simulink model "adc"  (R2024a)
settings: configuration reference "standardSILConfiguraitonParams" (kept outside this file)
undefined symbols (not defined in the file): stepSize_s
libraries: simulink x2, aerolibatmos2 x1
settings Model: Creator=GTAR  LastModifiedBy=jerem
settings ConfigSetRef: SourceName=standardSILConfiguraitonParams  SourceLocation=Base Workspace

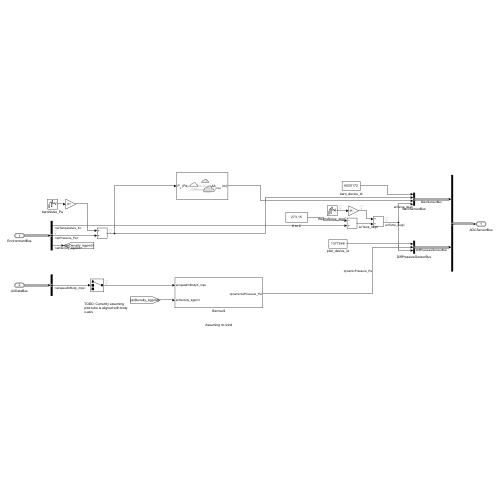
[thumbnail: Simulink's stored preview of the top-level diagram]
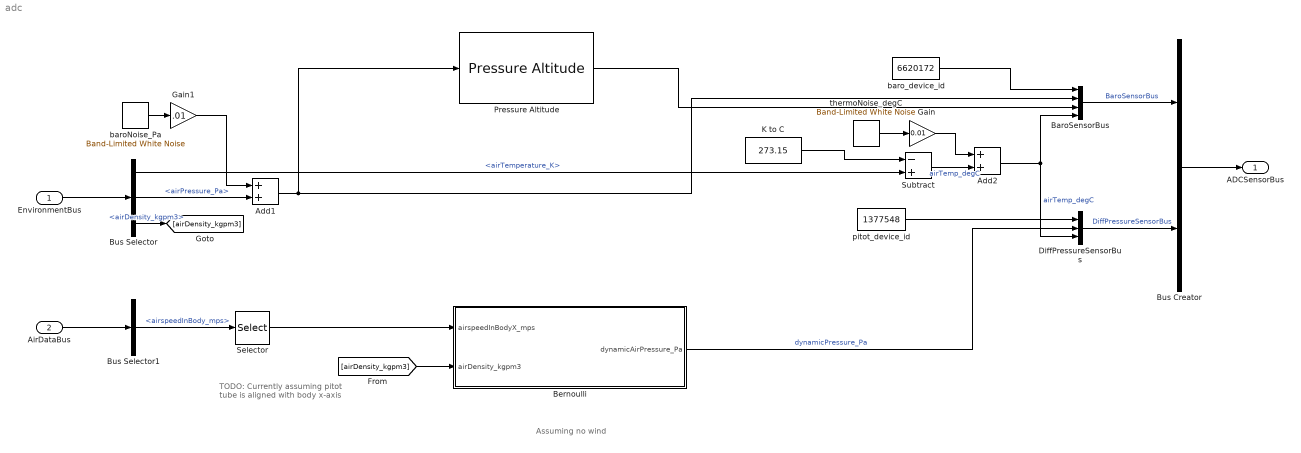
== system adc ==
  note: Assuming no wind
  note: TODO: Currently assuming pitot tube is aligned with body x-axis
  EnvironmentBus : Inport  OutDataTypeStr=Bus: EnvironmentBus
  AirDataBus : Inport  Port=2  OutDataTypeStr=Bus: AirData
  Add1 : Sum
  Add2 : Sum
  BaroSensorBus : BusCreator  Inputs=4  OutDataTypeStr=Bus: BaroSensorBus
      settings: InheritFromInputs=off
  Bernoulli : Subsystem
  Bus Creator : BusCreator  Inputs=2  OutDataTypeStr=Bus: ADCSensorBus
      settings: InheritFromInputs=off
  Bus Selector : BusSelector  OutputSignals=AirEnvironment.airTemperature_K,AirEnvironment.airPressure_Pa,AirEnvironment.airDensity_kgpm3
  Bus Selector1 : BusSelector  OutputSignals=airspeedInBody_mps
  DiffPressureSensorBus : BusCreator  Inputs=3  OutDataTypeStr=Bus: DiffPressureSensorBus
      settings: InheritFromInputs=off
  Gain : Gain  Gain=0.01
  Gain1 : Gain  Gain=.01
  K to C : Constant  Value=273.15
  Pressure Altitude : aerolibatmos2/Pressure Altitude  units=Metric (MKS)  action=Warning
  Selector : Selector  InputPortWidth=3  IndexOptions=Index vector (dialog)  Indices=1  OutputSizes=1
  Subtract : Sum  Inputs=-+
  baroNoise_Pa : simulink/Sources/Band-Limited White Noise  Cov=parameters.baro.noisePower_Pa  Ts=stepSize_s  seed=[23341]
  baro_device_id : Constant  Value=6620172  OutDataTypeStr=Inherit: Inherit via back propagation
  pitot_device_id : Constant  Value=1377548  OutDataTypeStr=Inherit: Inherit via back propagation
  thermoNoise_degC : simulink/Sources/Band-Limited White Noise  Cov=parameters.thermo.noisePower_degC  Ts=stepSize_s  seed=[23341]
  ADCSensorBus : Outport  OutDataTypeStr=Bus: ADCSensorBus
  wires:
  AirDataBus/1 -> Bus Selector1/1
  EnvironmentBus/1 -> Bus Selector/1
  Add2/1 -> BaroSensorBus/4, DiffPressureSensorBus/3  "airTemp_degC"
  Bus Selector1/1 -> Selector/1  "<airspeedInBody_mps>"
  K to C/1 -> Subtract/1
  Bus Selector/1 -> Subtract/2  "<airTemperature_K>"
  baro_device_id/1 -> BaroSensorBus/1
  DiffPressureSensorBus/1 -> Bus Creator/2  "DiffPressureSensorBus"
  BaroSensorBus/1 -> Bus Creator/1  "BaroSensorBus"
  Bus Creator/1 -> ADCSensorBus/1
  pitot_device_id/1 -> DiffPressureSensorBus/1
  Add1/1 -> BaroSensorBus/2, Pressure Altitude/1
  Bernoulli/1(dynamicAirPressure_Pa) -> DiffPressureSensorBus/2  "dynamicPressure_Pa"
  Bus Selector/2 -> Add1/2  "<airPressure_Pa>"
  baroNoise_Pa/1 -> Gain1/1
  Subtract/1 -> Add2/2  "airTemp_degC"
  Gain/1 -> Add2/1
  Selector/1 -> Bernoulli/1(airspeedInBodyX_mps)
  thermoNoise_degC/1 -> Gain/1
  Pressure Altitude/1 -> BaroSensorBus/3
  Bus Selector/3 -> [airDensity_kgpm3]  "<airDensity_kgpm3>"
  [airDensity_kgpm3] -> Bernoulli/2(airDensity_kgpm3)
  Gain1/1 -> Add1/1

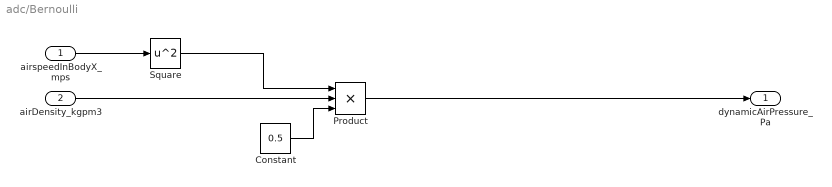
== system adc/Bernoulli ==
  airspeedInBodyX_mps : Inport
  airDensity_kgpm3 : Inport  Port=2
  Constant : Constant  Value=0.5
  Product : Product  Inputs=3
  Square : Math  Operator=square
  dynamicAirPressure_Pa : Outport
  wires:
  airspeedInBodyX_mps/1 -> Square/1
  Square/1 -> Product/1
  airDensity_kgpm3/1 -> Product/2
  Constant/1 -> Product/3
  Product/1 -> dynamicAirPressure_Pa/1
